simulink model "model"  (Simulink 7.9)
settings: Solver=ode45  StartTime=0.0  StopTime=10.0  RelTol=1e-3
libraries: simulink x8
settings Model: Creator=Mihail  LastModifiedBy=Mihail

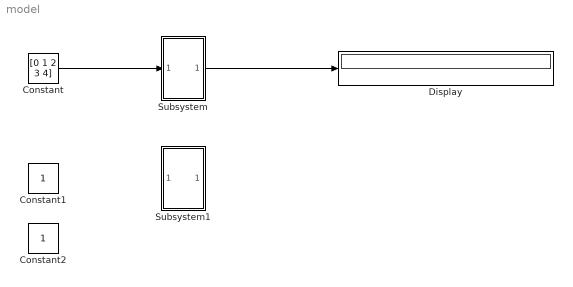
== system model ==
  Constant : Constant  Value=[0 1 2 3 4]
  Constant1 : Constant
  Constant2 : Constant
  Display : Display
  Subsystem : Subsystem
  Subsystem1 : Subsystem
  wires:
  Subsystem/1(Out1) -> Display/1
  Constant/1 -> Subsystem/1(In1)

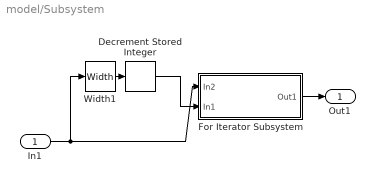
== system model/Subsystem ==
  In1 : Inport
  Decrement Stored Integer : simulink/Additional Math & Discrete/Additional Math: Increment - Decrement/Decrement Stored Integer
  For Iterator Subsystem : Subsystem  TreatAsAtomicUnit=on
  Width1 : Width  DataType=int8
  Out1 : Outport
  wires:
  In1/1 -> Width1/1, For Iterator Subsystem/1(In2)
  Width1/1 -> Decrement Stored Integer/1
  Decrement Stored Integer/1 -> For Iterator Subsystem/2(In1)
  For Iterator Subsystem/1(Out1) -> Out1/1

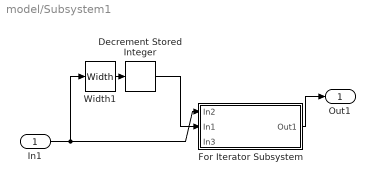
== system model/Subsystem1 ==
  In1 : Inport
  Decrement Stored Integer : simulink/Additional Math & Discrete/Additional Math: Increment - Decrement/Decrement Stored Integer
  For Iterator Subsystem : Subsystem  TreatAsAtomicUnit=on
  Width1 : Width  DataType=int8
  Out1 : Outport
  wires:
  For Iterator Subsystem/1(Out1) -> Out1/1
  Decrement Stored Integer/1 -> For Iterator Subsystem/2(In1)
  Width1/1 -> Decrement Stored Integer/1
  In1/1 -> For Iterator Subsystem/1(In2), Width1/1

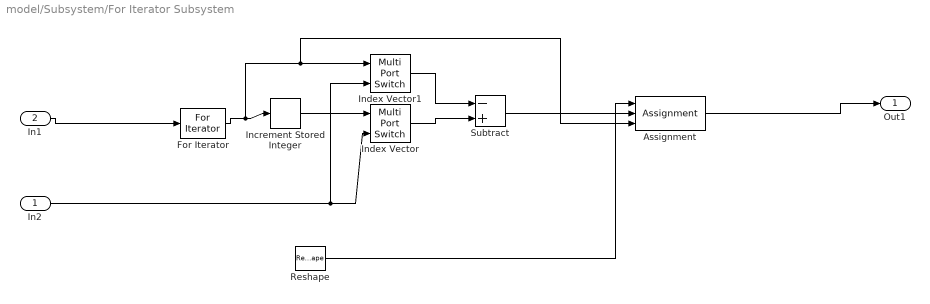
== system model/Subsystem/For Iterator Subsystem ==
  In2 : Inport
  In1 : Inport  Port=2
  Assignment : Assignment  IndexOptions=Index vector (port)  Indices=1  OutputSizes=1
  For Iterator : ForIterator  ResetStates=reset  IterationSource=external
  Increment Stored Integer : simulink/Additional Math & Discrete/Additional Math: Increment - Decrement/Increment Stored Integer
  Index Vector : MultiPortSwitch  Inputs=1  zeroidx=off
  Index Vector1 : MultiPortSwitch  Inputs=1  zeroidx=off
  Reshape : Reshape  OutputDimensionality=Customize  OutputDimensions=[1,4]
  Subtract : Sum  Inputs=-+
  Out1 : Outport
  wires:
  For Iterator/1 -> Increment Stored Integer/1, Index Vector1/1, Assignment/3
  Increment Stored Integer/1 -> Index Vector/1
  In1/1 -> For Iterator/1
  In2/1 -> Index Vector/2, Index Vector1/2
  Index Vector1/1 -> Subtract/1
  Index Vector/1 -> Subtract/2
  Subtract/1 -> Assignment/2
  Assignment/1 -> Out1/1
  Reshape/1 -> Assignment/1

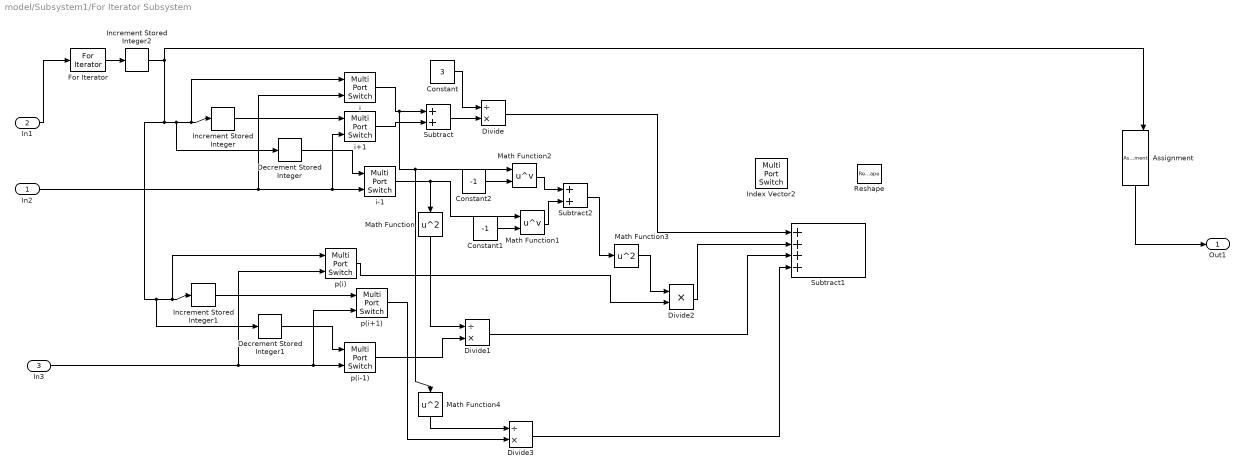
== system model/Subsystem1/For Iterator Subsystem ==
  In2 : Inport
  In1 : Inport  Port=2
  In3 : Inport  Port=3
  Assignment : Assignment  IndexOptions=Index vector (port)  Indices=1  OutputSizes=1
  Constant : Constant  Value=3
  Constant1 : Constant  Value=-1
  Constant2 : Constant  Value=-1
  Decrement Stored Integer : simulink/Additional Math & Discrete/Additional Math: Increment - Decrement/Decrement Stored Integer
  Decrement Stored Integer1 : simulink/Additional Math & Discrete/Additional Math: Increment - Decrement/Decrement Stored Integer
  Divide : Product  Inputs=/*
  Divide1 : Product  Inputs=/*
  Divide2 : Product  Inputs=**
  Divide3 : Product  Inputs=/*
  For Iterator : ForIterator  ResetStates=reset  IterationSource=external
  Increment Stored Integer : simulink/Additional Math & Discrete/Additional Math: Increment - Decrement/Increment Stored Integer
  Increment Stored Integer1 : simulink/Additional Math & Discrete/Additional Math: Increment - Decrement/Increment Stored Integer
  Increment Stored Integer2 : simulink/Additional Math & Discrete/Additional Math: Increment - Decrement/Increment Stored Integer
  Index Vector2 : MultiPortSwitch  Inputs=1  zeroidx=off
  Math Function : Math  Operator=square  SaturateOnIntegerOverflow=on
  Math Function1 : Math  Operator=pow  SaturateOnIntegerOverflow=on
  Math Function2 : Math  Operator=pow  SaturateOnIntegerOverflow=on
  Math Function3 : Math  Operator=square  SaturateOnIntegerOverflow=on
  Math Function4 : Math  Operator=square  SaturateOnIntegerOverflow=on
  Reshape : Reshape  OutputDimensionality=Customize  OutputDimensions=[1,5]
  Subtract : Sum
  Subtract1 : Sum  Inputs=++++
  Subtract2 : Sum
  i : MultiPortSwitch  Inputs=1  zeroidx=off
  i+1 : MultiPortSwitch  Inputs=1  zeroidx=off
  i-1 : MultiPortSwitch  Inputs=1  zeroidx=off
  p(i) : MultiPortSwitch  Inputs=1  zeroidx=off
  p(i+1) : MultiPortSwitch  Inputs=1  zeroidx=off
  p(i-1) : MultiPortSwitch  Inputs=1  zeroidx=off
  Out1 : Outport
  wires:
  Assignment/1 -> Out1/1
  i+1/1 -> Subtract/2
  i/1 -> Subtract/1, Math Function2/1, Math Function4/1
  In2/1 -> i/2, i+1/2, i-1/2
  In1/1 -> For Iterator/1
  Increment Stored Integer/1 -> i+1/1
  For Iterator/1 -> Increment Stored Integer2/1
  Decrement Stored Integer/1 -> i-1/1
  Subtract/1 -> Divide/2
  Constant/1 -> Divide/1
  In3/1 -> p(i)/2, p(i+1)/2, p(i-1)/2
  Increment Stored Integer1/1 -> p(i+1)/1
  Decrement Stored Integer1/1 -> p(i-1)/1
  p(i-1)/1 -> Divide1/2
  i-1/1 -> Math Function/1, Math Function1/1
  Math Function/1 -> Divide1/1
  Divide/1 -> Subtract1/1
  Constant1/1 -> Math Function1/2
  Constant2/1 -> Math Function2/2
  Math Function2/1 -> Subtract2/1
  Math Function1/1 -> Subtract2/2
  Subtract2/1 -> Math Function3/1
  Math Function3/1 -> Divide2/1
  p(i)/1 -> Divide2/2
  Divide2/1 -> Subtract1/2
  Math Function4/1 -> Divide3/1
  Divide1/1 -> Subtract1/3
  p(i+1)/1 -> Divide3/2
  Divide3/1 -> Subtract1/4
  Increment Stored Integer2/1 -> Increment Stored Integer/1, i/1, Decrement Stored Integer/1, Increment Stored Integer1/1, p(i)/1, Decrement Stored Integer1/1, Assignment/3
